simulink model "sm_potters_wheel"  (R2021b)
settings: Solver=ode15s  StartTime=0.0  StopTime=20  MaxStep=0.02  RelTol=1e-3  EnableMultiTasking=on
model workspace: external: MATLAB File sm_potters_wheel_params.m (data not in the file)
undefined symbols (not defined in the file or in its folder): actuation, clay, floor, leg, marker, shaft, sigbuilder_block, tabletop, wheel, X, Y, Z
libraries: sm_lib x48, nesl_utility x11
(part 1 of 2)
Description:
  | Sensing Composite Forces and Torques in Joints - Potter's Wheel
  | 
  | The example shows how you can sense forces and torques acting at joints. A
  | potter's wheel spins with a piecewise linear velocity profile while holding a piece
  | of clay off center. The clay creates a dynamic imbalance, generating periodic
  | constraint forces at the joints. Viscous damping accounts for energy dissipation
  | in the axle.
  | 
  | Scopes 1 and 2 show the composite forces and torques that you can sense at
  | the joints. These include the constraint forces and torques and also the total
  | forces and torques, which are the net sum of constraint, actuation and internal
  | components. The constraint components are zero in the direction of motion,
  | while the actuation and internal components are zero in the constrained directions.
  | 
  | If a multibody system is overconstrained, Simscape Multibody(TM) distributes the
  | constraint forces and torques over the joints enforcing the redundant constraints.
  | The vertical constraint forces acting at the leg weld joints are one example.
  | These forces, shown in Scope 3, add up to the total weight of the table. They
  | are nearly equal, with only slight discrepancies among them due to asymmetries
  | in the shape and position of the clay.
settings Model: Creator=The MathWorks, Inc.  LastModifiedBy=The MathWorks, Inc.
settings SolverCC: AlgebraicLoopSolver=TrustRegion
settings DataIOCC: LimitDataPoints=on  SaveFormat=Array  ReturnWorkspaceOutputs=off
settings OptimizationCC: LifeSpan=inf
settings DebuggingCC: SolverPrmCheckMsg=warning  SFUnexpectedBacktrackingDiag=warning  SFNoUnconditionalDefaultTransitionDiag=warning  SFExecutionAtInitializationDiag=none  SFMachineParentedDataDiag=warning  ArithmeticOperatorsInVariantConditions=warning
settings HardwareCC: ProdBitPerPointer=32  ProdBitPerSizeT=32  ProdBitPerPtrDiffT=32  ProdLargestAtomicFloat=None  ProdIntDivRoundTo=Undefined  ProdEndianess=Unspecified  ProdWordSize=32  ProdHWDeviceType=32-bit Generic
settings ModelReferenceCC: PropagateSignalLabelsOutOfModel=off
settings SFSimCC: SimUseLocalCustomCode=off  CustomCodeUndefinedFunction=UseInterfaceOnly
settings RTWCC: RTWUseLocalCustomCode=off
settings CodeAppCC: StateflowObjectComments=on
settings GRTTargetCC: TargetLangStandard=C89/C90 (ANSI)
settings ConfigComp: CovMetricSettings=dw  CovSaveCumulativeToWorkspaceVar=on  CovSaveSingleToWorkspaceVar=on  CovExternalEMLEnable=off  CovSFcnEnable=off
settings SimscapeCC: SimscapeNormalizeSystem=off
settings ConfigurationSet: Description=SimMechanics 2G
settings ExplorerConfigSet: InternalSimMechanicsExplorerSettings="<ExplorerConfiguration><canonicalview>default</canonicalview><AnimationSetting><BasePlaybackSpeed>1.0</BasePlaybackSpeed><PlaybackSpeedFactor>1.0</PlaybackSpeedFactor></AnimationSetting><TilePanel><TileInfo><Tiles Columns=\"1\" Count=\"1\" Rows=\"1\"><Column Left=\"2\" Weight=\"1\"/><Column Left=\"697\"/><Row Top=\"2\" Weight=\"1\"/><Row Top=\"673\"/><Tile Height=\"1\" Width=\"1\" X=\"0\" Y=\"0\"/></Tiles></TileInfo><SceneInfo><SceneViewer><BGColor><R>0.91372549533843994</R><G>0.92941176891326904</G><B>0.92941176891326904</B></BGColor><Camera><Position><X>1.1996229894546588</X><Y>-1.226238345212963</Y><Z>1.5340072938881431</Z></Position><Center><X>-0.0094998831543196653</X><Y>-0.017115472603984407</Y><Z>0.32488442127917233</Z></Center><Up><X>-0.40824829046386307</X><Y>0.40824829046386307</Y><Z>0.81649658092772615</Z></Up><Left>-0.60569783977149305</Left><Right>0.60569783977149305</Right><Bottom>-0.53853769779510163</Bottom><Top>0.53853769779510163</Top></Camera></SceneViewer></SceneInfo></TilePanel></ExplorerConfiguration>"

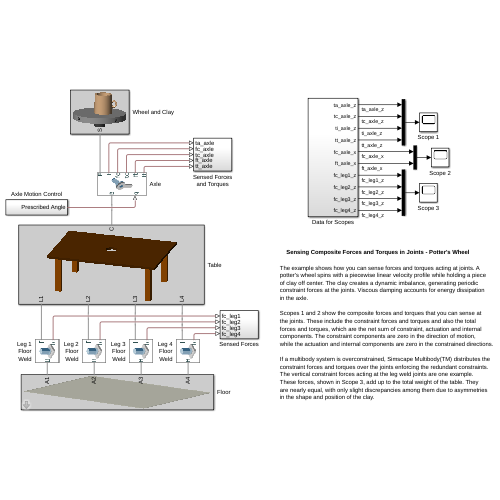
[thumbnail: Simulink's stored preview of the top-level diagram]
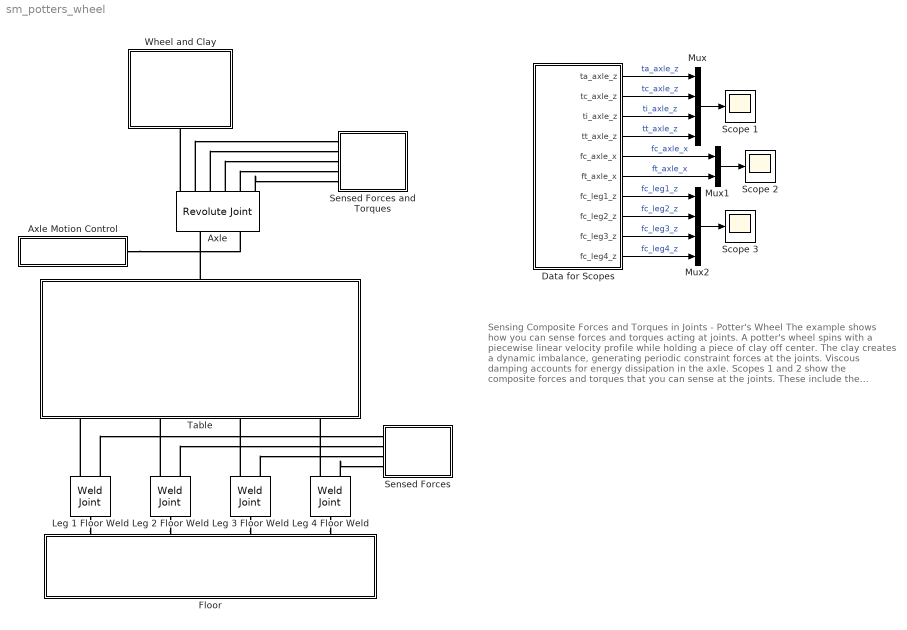
== system sm_potters_wheel ==
  note: Sensing Composite Forces and Torques in Joints - Potter's Wheel
      |
      | The example shows how you can sense forces and torques acting at joints. A
      | potter's wheel spins with a piecewise linear velocity profile while holding a piece
      | of clay off center. The clay creates a dynamic imbalance, generating periodic
      | constraint forces at the joints. Viscous damping accounts for energy dissipation
      | in the axle.
      |
      | Scopes 1 and 2 show the composite forces and torques that you can sense at
      | the joints. These include the constraint forces and torques and also the total
      | forces and torques, which are the net sum of constraint, actuation and internal
      | components. The constraint components are zero in the direction of motion,
      | while the actuation and internal components are zero in the constrained directions.
      |
      | If a multibody system is overconstrained, Simscape Multibody(TM) distributes the
      | constraint forces and torques over the joints enforcing the redundant constraints.
      | The vertical constraint forces acting at the leg weld joints are one example.
      | These forces, shown in Scope 3, add up to the total weight of the table. They
      | are nearly equal, with only slight discrepancies among them due to asymmetries
      | in the shape and position of the clay.
  Axle : sm_lib/Joints/Revolute Joint  JointMode=Normal  SenseConstraintForce=on  SenseConstraintForceX=off  SenseConstraintForceY=off  SenseConstraintForceZ=off  SenseConstraintTorque=on  SenseConstraintTorqueX=off  SenseConstraintTorqueY=off  SenseConstraintTorqueZ=off  SenseTotalForce=on  SenseTotalForceX=off  SenseTotalForceY=off  SenseTotalForceZ=off  SenseTotalTorque=on  SenseTotalTorqueX=off  SenseTotalTorqueY=off  SenseTotalTorqueZ=off  CompositeWrenchDir=BaseOnFollower  CompositeWrenchFrame=BaseFrame  EquilibriumPosition=0  EquilibriumPositionUnits=deg  SpringStiffness=0  SpringStiffnessUnits=N*m/deg  DampingCoefficient=axle.R.damping  DampingCoefficientUnits=N*m/(deg/s)  TorqueActuationMode=ComputedTorque  MotionActuationMode=InputMotion  SensePosition=off  SenseVelocity=off  SenseAcceleration=off  SenseTorqueForce=on  SenseLowerLimitTorqueForce=off  SenseUpperLimitTorqueForce=off  LowerLimitSpecify=off  LowerLimitBound=-90  LowerLimitBoundUnits=deg  LowerLimitStiffness=1e4  LowerLimitStiffnessUnits=N*m/deg  LowerLimitDamping=10  LowerLimitDampingUnits=N*m/(deg/s)  LowerLimitTransitionRegionWidth=0.1  LowerLimitTransitionRegionWidthUnits=deg  UpperLimitSpecify=off  UpperLimitBound=90  UpperLimitBoundUnits=deg  UpperLimitStiffness=1e4  UpperLimitStiffnessUnits=N*m/deg  UpperLimitDamping=10  UpperLimitDampingUnits=N*m/(deg/s)  UpperLimitTransitionRegionWidth=0.1  UpperLimitTransitionRegionWidthUnits=deg  PositionTargetSpecify=off  PositionTargetPriority=High  PositionTargetValue=0  PositionTargetValueUnits=deg  VelocityTargetSpecify=off  VelocityTargetPriority=High  VelocityTargetValue=0  VelocityTargetValueUnits=deg/s
  Axle Motion Control : Subsystem
  Data for Scopes : Subsystem
  Floor : Subsystem  mask(Floor){l=floor.length, w=floor.width, t=floor.thickness, la=tabletop.length - 2*tabletop.legoffset, wa=tabletop.width - 2*tabletop.legoffset, color=floor.color}
      mask prompts: l "Length (cm)"; w "Width (cm)"; t "Thickness (cm)"; la "Anchor Point Rectangle Length (cm)"; wa "Anchor Point Rectangle Width (cm)"; color "Color (RGB)"
      mask help:
      | This block models a floor for a table to stand on.
      |
      | Ports A1, A2, A3 and A4 correspond to four anchor frames on the upper plane of the floor. They lie at the corners of a rectangle aligned with the X and Y directions.
      mask init:
      | % Coordinates of anchor points
      | xa = la/2;
      | ya = wa/2;
      mask DialogControl Container4 Prompt: Dimensions
      mask DialogControl Container5 Prompt: Material Properties
      mask Display:
      | image(fullfile(matlabroot,'toolbox','physmod','sm','smdemos','potters_wheel','images','sm_pwheel_floor.png'));
      | port_label('RConn', 1, 'A1');
      | port_label('RConn', 2, 'A2');
      | port_label('RConn', 3, 'A3');
      | port_label('RConn', 4, 'A4');
  Leg 1 Floor Weld : sm_lib/Joints/Weld Joint  JointMode=Normal  SenseConstraintForce=on  SenseConstraintForceX=off  SenseConstraintForceY=off  SenseConstraintForceZ=off  SenseConstraintTorque=off  SenseConstraintTorqueX=off  SenseConstraintTorqueY=off  SenseConstraintTorqueZ=off  SenseTotalForce=off  SenseTotalForceX=off  SenseTotalForceY=off  SenseTotalForceZ=off  SenseTotalTorque=off  SenseTotalTorqueX=off  SenseTotalTorqueY=off  SenseTotalTorqueZ=off  CompositeWrenchDir=BaseOnFollower  CompositeWrenchFrame=BaseFrame
  Leg 2 Floor Weld : sm_lib/Joints/Weld Joint  JointMode=Normal  SenseConstraintForce=on  SenseConstraintForceX=off  SenseConstraintForceY=off  SenseConstraintForceZ=off  SenseConstraintTorque=off  SenseConstraintTorqueX=off  SenseConstraintTorqueY=off  SenseConstraintTorqueZ=off  SenseTotalForce=off  SenseTotalForceX=off  SenseTotalForceY=off  SenseTotalForceZ=off  SenseTotalTorque=off  SenseTotalTorqueX=off  SenseTotalTorqueY=off  SenseTotalTorqueZ=off  CompositeWrenchDir=BaseOnFollower  CompositeWrenchFrame=BaseFrame
  Leg 3 Floor Weld : sm_lib/Joints/Weld Joint  JointMode=Normal  SenseConstraintForce=on  SenseConstraintForceX=off  SenseConstraintForceY=off  SenseConstraintForceZ=off  SenseConstraintTorque=off  SenseConstraintTorqueX=off  SenseConstraintTorqueY=off  SenseConstraintTorqueZ=off  SenseTotalForce=off  SenseTotalForceX=off  SenseTotalForceY=off  SenseTotalForceZ=off  SenseTotalTorque=off  SenseTotalTorqueX=off  SenseTotalTorqueY=off  SenseTotalTorqueZ=off  CompositeWrenchDir=BaseOnFollower  CompositeWrenchFrame=BaseFrame
  Leg 4 Floor Weld : sm_lib/Joints/Weld Joint  JointMode=Normal  SenseConstraintForce=on  SenseConstraintForceX=off  SenseConstraintForceY=off  SenseConstraintForceZ=off  SenseConstraintTorque=off  SenseConstraintTorqueX=off  SenseConstraintTorqueY=off  SenseConstraintTorqueZ=off  SenseTotalForce=off  SenseTotalForceX=off  SenseTotalForceY=off  SenseTotalForceZ=off  SenseTotalTorque=off  SenseTotalTorqueX=off  SenseTotalTorqueY=off  SenseTotalTorqueZ=off  CompositeWrenchDir=BaseOnFollower  CompositeWrenchFrame=BaseFrame
  Mux : Mux
  Mux1 : Mux  Inputs=2
  Mux2 : Mux
  Scope 1 : Scope
  Scope 2 : Scope
  Scope 3 : Scope
  Sensed Forces : Subsystem
  Sensed Forces and Torques : Subsystem
  Table : Subsystem  mask(Table){}
      mask Display:
      | image(fullfile(matlabroot,'toolbox','physmod','sm','smdemos','potters_wheel','images','sm_pwheel_table.png'));
      | port_label('LConn', 1, 'L1')
      | port_label('LConn', 2, 'L2')
      | port_label('LConn', 3, 'L3')
      | port_label('LConn', 4, 'L4')
      | port_label('RConn', 1, 'C')
  Wheel and Clay : Subsystem  mask(Wheel and Clay){}
      mask Display:
      | image(fullfile(matlabroot,'toolbox','physmod','sm','smdemos','potters_wheel','images','sm_pwheel_wheelandclay.png'));
      | port_label('LConn', 1, 'S');
  wires:
  Mux/1 -> Scope 1/1
  Mux2/1 -> Scope 3/1
  Data for Scopes/1(ta_axle_z) -> Mux/1  "ta_axle_z"
  Data for Scopes/2(tc_axle_z) -> Mux/2  "tc_axle_z"
  Data for Scopes/3(ti_axle_z) -> Mux/3  "ti_axle_z"
  Data for Scopes/4(tt_axle_z) -> Mux/4  "tt_axle_z"
  Data for Scopes/5(fc_axle_x) -> Mux1/1  "fc_axle_x"
  Data for Scopes/6(ft_axle_x) -> Mux1/2  "ft_axle_x"
  Mux1/1 -> Scope 2/1
  Data for Scopes/8(fc_leg2_z) -> Mux2/2  "fc_leg2_z"
  Data for Scopes/9(fc_leg3_z) -> Mux2/3  "fc_leg3_z"
  Data for Scopes/10(fc_leg4_z) -> Mux2/4  "fc_leg4_z"
  Data for Scopes/7(fc_leg1_z) -> Mux2/1  "fc_leg1_z"
  connections:
  Axle/RConn1 -- Wheel and Clay/LConn1
  Table/RConn1 -- Axle/LConn1
  Axle Motion Control/RConn1 -- Axle/LConn2
  Axle/RConn6 -- Sensed Forces and Torques/LConn5
  Axle/RConn5 -- Sensed Forces and Torques/LConn4
  Axle/RConn4 -- Sensed Forces and Torques/LConn3
  Axle/RConn3 -- Sensed Forces and Torques/LConn2
  Axle/RConn2 -- Sensed Forces and Torques/LConn1
  Leg 1 Floor Weld/LConn1 -- Floor/RConn1
  Leg 1 Floor Weld/RConn1 -- Table/LConn1
  Leg 2 Floor Weld/LConn1 -- Floor/RConn2
  Leg 2 Floor Weld/RConn1 -- Table/LConn2
  Leg 3 Floor Weld/RConn1 -- Table/LConn3
  Leg 3 Floor Weld/LConn1 -- Floor/RConn3
  Leg 4 Floor Weld/RConn1 -- Table/LConn4
  Leg 4 Floor Weld/LConn1 -- Floor/RConn4
  Leg 4 Floor Weld/RConn2 -- Sensed Forces/LConn4
  Leg 3 Floor Weld/RConn2 -- Sensed Forces/LConn3
  Leg 2 Floor Weld/RConn2 -- Sensed Forces/LConn2
  Leg 1 Floor Weld/RConn2 -- Sensed Forces/LConn1

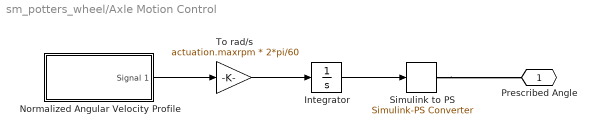
== system sm_potters_wheel/Axle Motion Control ==
  Integrator : Integrator
  Normalized Angular Velocity Profile : Subsystem  Tag=STV Subsys  LoadFcn=sigbuilder_block('load');  StartFcn=sigbuilder_block('start');  StopFcn=sigbuilder_block('stop');  ClipboardFcn=sigbuilder_block('clipboard');  mask(Sigbuilder block){tuvar=[0:10]}
      mask help: Simulink:masks:SigbuilderBlock_MD
      mask init:
      | if ~strcmp(get_param(bdroot(gcbh),'SimulationStatus'),'stopped') tuvar = sigbuilder_block('maskInit'); end
      settings: CopyFcn=sigbuilder_block('copy');  DeleteFcn=sigbuilder_block('delete');  ModelCloseFcn=sigbuilder_block('modelClose');  PreSaveFcn=sigbuilder_block('preSave');  PauseFcn=sigbuilder_block('pause');  ContinueFcn=sigbuilder_block('continue');  NameChangeFcn=sigbuilder_block('namechange');  OpenFcn=sigbuilder_block('open',[437.6 199.2 550.4 400 ]);  CloseFcn=sigbuilder_block('close');
      mask Display: plot(0, 0, 100, 100,[2, 2, 32, 32, 2], [68, 8, 8, 68, 68],[32, 2], [38, 38], [32, 19, 2],[53, 60, 44], [32, 17, 17, 2],[16, 16, 31, 31]);txt = getActiveGroup(gcbh);text(2, 100, txt,'verticalAlignment', 'top');
  Simulink to PS : nesl_utility/Simulink-PS Converter  PhysicalDomain=network_engine_domain  SubClassName=ps_input  LeftPortType=input  RightPortType=output  PseudoPeriodic=off  Frequencies=[]  NoiseDistribution=none  NoiseParameters=[]  Unit=rad  AffineConversion=off  FilteringAndDerivatives=filter  SimscapeFilterOrder=2  InputFilterTimeConstant=0.1  UdotUserProvided=1
      settings: SourceProductBaseCode=PW,SS
  To rad/s : Gain  Gain=actuation.maxrpm * 2*pi/60
  Prescribed Angle : PMIOPort  Side=Right
  wires:
  Normalized Angular Velocity Profile/1(Signal 1) -> To rad/s/1
  To rad/s/1 -> Integrator/1
  Integrator/1 -> Simulink to PS/1
  connections:
  Simulink to PS/RConn1 -- Prescribed Angle/RConn1

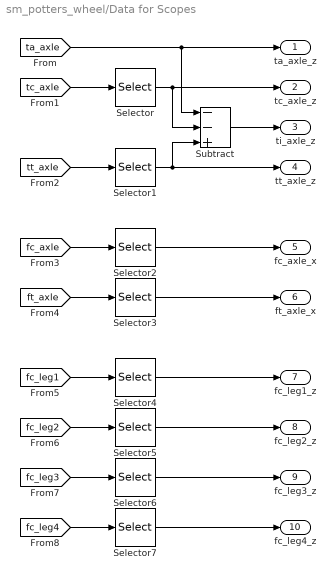
== system sm_potters_wheel/Data for Scopes ==
  Selector : Selector  InputPortWidth=3  IndexOptions=Index vector (dialog)  Indices=3  OutputSizes=1
  Selector1 : Selector  InputPortWidth=3  IndexOptions=Index vector (dialog)  Indices=3  OutputSizes=1
  Selector2 : Selector  InputPortWidth=3  IndexOptions=Index vector (dialog)  Indices=1  OutputSizes=1
  Selector3 : Selector  InputPortWidth=3  IndexOptions=Index vector (dialog)  Indices=1  OutputSizes=1
  Selector{4..7} (4 alike) : Selector  InputPortWidth=3  IndexOptions=Index vector (dialog)  Indices=3  OutputSizes=3
  Subtract : Sum  Inputs=--+
  ta_axle_z : Outport
  tc_axle_z : Outport  Port=2
  ti_axle_z : Outport  Port=3
  tt_axle_z : Outport  Port=4
  fc_axle_x : Outport  Port=5
  ft_axle_x : Outport  Port=6
  fc_leg1_z : Outport  Port=7
  fc_leg2_z : Outport  Port=8
  fc_leg3_z : Outport  Port=9
  fc_leg4_z : Outport  Port=10
  wires:
  [fc_leg1] -> Selector4/1
  [fc_axle] -> Selector2/1
  Selector/1 -> tc_axle_z/1, Subtract/2
  [tt_axle] -> Selector1/1
  [ft_axle] -> Selector3/1
  [tc_axle] -> Selector/1
  [ta_axle] -> ta_axle_z/1, Subtract/1
  Selector1/1 -> tt_axle_z/1, Subtract/3
  Subtract/1 -> ti_axle_z/1
  Selector4/1 -> fc_leg1_z/1
  Selector2/1 -> fc_axle_x/1
  Selector3/1 -> ft_axle_x/1
  [fc_leg2] -> Selector5/1
  Selector5/1 -> fc_leg2_z/1
  [fc_leg3] -> Selector6/1
  Selector6/1 -> fc_leg3_z/1
  [fc_leg4] -> Selector7/1
  Selector7/1 -> fc_leg4_z/1

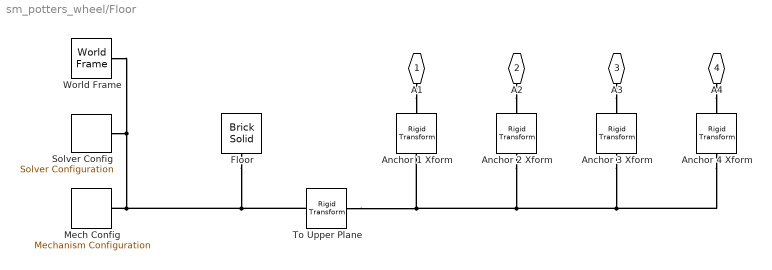
== system sm_potters_wheel/Floor ==
  Anchor 1 Xform : sm_lib/Frames and Transforms/Rigid Transform  TranslationMethod=Cartesian  TranslationStandardOffset=0  TranslationLengthUnit=cm  TranslationStandardAxis=+Z  TranslationCartesianOffset=[-xa ya 0]  TranslationROffset=0  TranslationROffsetUnits=m  TranslationZOffset=0  TranslationZOffsetUnits=m  TranslationThetaOffset=0  TranslationThetaOffsetUnits=deg  RotationMethod=None  RotationAngleUnits=deg  RotationStandardAxis=+Z  RotationAngle=0.0  RotationArbitraryAxis=[0 0 1]  FollAlignAxisA=+X  BaseAlignAxisA=+Y  FollAlignAxisB=+Y  BaseAlignAxisB=+Z  RotationSequenceAxes=FollowerAxes  RotationSequence=XYX  RotationSequenceAngles=[0 0 0]  RotationSequenceAnglesUnits=deg  RotationMatrix=[1 0 0; 0 1 0; 0 0 1]
  Anchor 2 Xform : sm_lib/Frames and Transforms/Rigid Transform  TranslationMethod=Cartesian  TranslationStandardOffset=0  TranslationLengthUnit=cm  TranslationStandardAxis=+Z  TranslationCartesianOffset=[-xa -ya 0]  TranslationROffset=0  TranslationROffsetUnits=m  TranslationZOffset=0  TranslationZOffsetUnits=m  TranslationThetaOffset=0  TranslationThetaOffsetUnits=deg  RotationMethod=None  RotationAngleUnits=deg  RotationStandardAxis=+Z  RotationAngle=0.0  RotationArbitraryAxis=[0 0 1]  FollAlignAxisA=+X  BaseAlignAxisA=+Y  FollAlignAxisB=+Y  BaseAlignAxisB=+Z  RotationSequenceAxes=FollowerAxes  RotationSequence=XYX  RotationSequenceAngles=[0 0 0]  RotationSequenceAnglesUnits=deg  RotationMatrix=[1 0 0; 0 1 0; 0 0 1]
  Anchor 3 Xform : sm_lib/Frames and Transforms/Rigid Transform  TranslationMethod=Cartesian  TranslationStandardOffset=0  TranslationLengthUnit=cm  TranslationStandardAxis=+Z  TranslationCartesianOffset=[xa -ya 0]  TranslationROffset=0  TranslationROffsetUnits=m  TranslationZOffset=0  TranslationZOffsetUnits=m  TranslationThetaOffset=0  TranslationThetaOffsetUnits=deg  RotationMethod=None  RotationAngleUnits=deg  RotationStandardAxis=+Z  RotationAngle=0.0  RotationArbitraryAxis=[0 0 1]  FollAlignAxisA=+X  BaseAlignAxisA=+Y  FollAlignAxisB=+Y  BaseAlignAxisB=+Z  RotationSequenceAxes=FollowerAxes  RotationSequence=XYX  RotationSequenceAngles=[0 0 0]  RotationSequenceAnglesUnits=deg  RotationMatrix=[1 0 0; 0 1 0; 0 0 1]
  Anchor 4 Xform : sm_lib/Frames and Transforms/Rigid Transform  TranslationMethod=Cartesian  TranslationStandardOffset=0  TranslationLengthUnit=cm  TranslationStandardAxis=+Z  TranslationCartesianOffset=[xa ya 0]  TranslationROffset=0  TranslationROffsetUnits=m  TranslationZOffset=0  TranslationZOffsetUnits=m  TranslationThetaOffset=0  TranslationThetaOffsetUnits=deg  RotationMethod=None  RotationAngleUnits=deg  RotationStandardAxis=+Z  RotationAngle=0.0  RotationArbitraryAxis=[0 0 1]  FollAlignAxisA=+X  BaseAlignAxisA=+Y  FollAlignAxisB=+Y  BaseAlignAxisB=+Z  RotationSequenceAxes=FollowerAxes  RotationSequence=XYX  RotationSequenceAngles=[0 0 0]  RotationSequenceAnglesUnits=deg  RotationMatrix=[1 0 0; 0 1 0; 0 0 1]
  Floor : sm_lib/Body Elements/Brick Solid  GraphicAmbientColor=[0.15 0.15 0.15 1.0]  BasedOnType=Density  BrickDimensions=[l w t]  BrickDimensionUnits=cm  CenterOfMass=[0 0 0]  CenterOfMassUnits=m  GraphicDiffuseColor=color  Density=1000  DensityUnits=kg/(m^3)  DoExposeReferenceFrame=on  GraphicEmissiveColor=[0.0 0.0 0.0 1.0]  ExportEntireGeometry=off  SerializedFrames=<Frames/>  MarkerShape=Sphere  MarkerSize=10  GraphicType=FromGeometry  InertiaType=PointMass  Mass=0  MassUnits=kg  MomentsOfInertia=[1 1 1]  MomentsOfInertiaUnits=kg*m^2  GraphicOpacity=0.5  ProductsOfInertia=[0 0 0]  ProductsOfInertiaUnits=kg*m^2  GraphicShininess=75  GraphicSpecularColor=[0.5 0.5 0.5 1.0]  GraphicVisPropType=SimpleVisualProperties
  Mech Config : sm_lib/Utilities/Mechanism Configuration  UniformGravity=Constant  GravityVector=[0 0 -9.80665]  GravityUnits=m/s^2  LinearizationDelta=0.001  JointModeTransitionNonlinearIterations=2
  Solver Config : nesl_utility/Solver Configuration  PhysicalDomain=network_engine_domain  SubClassName=solver  LeftPortType=input  RightPortType=generic  Tones=[]  Harmonics=[]  SimulateNoise=off  Profile=off  UseLocalSampling=off  EnableSwitchedLinearOptims=on  FrequencyDomain=off  UseCCode=off  RelTol=0.001  AbsTol=1e-06  MinStep=1e-09  ToWorkspace=off  RevertToSquareIcSolve=off  NumHomotopyIterations=100  PhasorMode=off  PhasorModeNumHarmonics=1  DoDC=off  ResidualTolerance=1e-09  UseLocalSolver=off  LocalSolverChoice=NE_BACKWARD_EULER_ADVANCER  LocalSolverSampleTime=0.001  DoFixedCost=off  MaxNonlinIter=3  MaxModeIter=2  ComputeImpulses=off  ImpulseIterations=2  LinearAlgebra=Sparse  EquationFormulation=NE_TIME_EF  DelaysMemoryBudget=1024  AutomaticFiltering=on  FilteringTimeConstant=0.001  PartitionStorageMethod=AS_NEEDED  PartitionMemoryBudget=1024  PartitionMethod=FAST
      settings: SourceProductBaseCode=PW,SS
  To Upper Plane : sm_lib/Frames and Transforms/Rigid Transform  TranslationMethod=Cartesian  TranslationStandardOffset=0  TranslationLengthUnit=cm  TranslationStandardAxis=+Z  TranslationCartesianOffset=[0 0 t/2]  TranslationROffset=0  TranslationROffsetUnits=m  TranslationZOffset=0  TranslationZOffsetUnits=m  TranslationThetaOffset=0  TranslationThetaOffsetUnits=deg  RotationMethod=None  RotationAngleUnits=deg  RotationStandardAxis=+Z  RotationAngle=0.0  RotationArbitraryAxis=[0 0 1]  FollAlignAxisA=+X  BaseAlignAxisA=+Y  FollAlignAxisB=+Y  BaseAlignAxisB=+Z  RotationSequenceAxes=FollowerAxes  RotationSequence=XYX  RotationSequenceAngles=[0 0 0]  RotationSequenceAnglesUnits=deg  RotationMatrix=[1 0 0; 0 1 0; 0 0 1]
  World Frame : sm_lib/Frames and Transforms/World Frame
  A1 : PMIOPort  Side=Right
  A2 : PMIOPort  Port=2  Side=Right
  A3 : PMIOPort  Port=3  Side=Right
  A4 : PMIOPort  Port=4  Side=Right
  connections:
  A2/RConn1 -- Anchor 2 Xform/RConn1
  A1/RConn1 -- Anchor 1 Xform/RConn1
  A3/RConn1 -- Anchor 3 Xform/RConn1
  A4/RConn1 -- Anchor 4 Xform/RConn1
  To Upper Plane/RConn1 -- Anchor 4 Xform/LConn1 -- Anchor 3 Xform/LConn1 -- Anchor 2 Xform/LConn1 -- Anchor 1 Xform/LConn1
  Solver Config/RConn1 -- Floor/RConn1 -- To Upper Plane/LConn1 -- Mech Config/RConn1 -- World Frame/RConn1

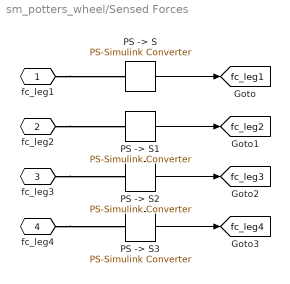
== system sm_potters_wheel/Sensed Forces ==
  PS -> S{,1..3} (4 alike) : nesl_utility/PS-Simulink Converter  PhysicalDomain=network_engine_domain  SubClassName=ps_output  LeftPortType=input  RightPortType=output  PseudoPeriodic=off  Frequencies=[]  Unit=N  AffineConversion=off
      settings: SourceProductBaseCode=PW,SS
  fc_leg1 : PMIOPort  Side=Left
  fc_leg2 : PMIOPort  Port=2  Side=Left
  fc_leg3 : PMIOPort  Port=3  Side=Left
  fc_leg4 : PMIOPort  Port=4  Side=Left
  tag scope: fc_leg1=global, fc_leg2=global, fc_leg3=global, fc_leg4=global
  wires:
  "PS -> S"/1 -> [fc_leg1]
  "PS -> S1"/1 -> [fc_leg2]
  "PS -> S2"/1 -> [fc_leg3]
  "PS -> S3"/1 -> [fc_leg4]
  connections:
  fc_leg1/RConn1 -- "PS -> S"/LConn1
  fc_leg2/RConn1 -- "PS -> S1"/LConn1
  fc_leg3/RConn1 -- "PS -> S2"/LConn1
  fc_leg4/RConn1 -- "PS -> S3"/LConn1

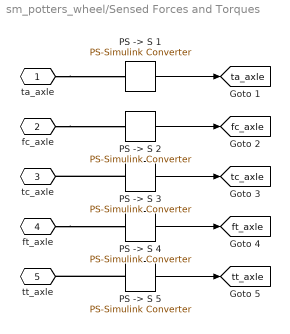
== system sm_potters_wheel/Sensed Forces and Torques ==
  "PS -> S 1" : nesl_utility/PS-Simulink Converter  PhysicalDomain=network_engine_domain  SubClassName=ps_output  LeftPortType=input  RightPortType=output  PseudoPeriodic=off  Frequencies=[]  Unit=N*m  AffineConversion=off
      settings: SourceProductBaseCode=PW,SS
  "PS -> S 2" : nesl_utility/PS-Simulink Converter  PhysicalDomain=network_engine_domain  SubClassName=ps_output  LeftPortType=input  RightPortType=output  PseudoPeriodic=off  Frequencies=[]  Unit=N  AffineConversion=off
      settings: SourceProductBaseCode=PW,SS
  "PS -> S 3" : nesl_utility/PS-Simulink Converter  PhysicalDomain=network_engine_domain  SubClassName=ps_output  LeftPortType=input  RightPortType=output  PseudoPeriodic=off  Frequencies=[]  Unit=N*m  AffineConversion=off
      settings: SourceProductBaseCode=PW,SS
  "PS -> S 4" : nesl_utility/PS-Simulink Converter  PhysicalDomain=network_engine_domain  SubClassName=ps_output  LeftPortType=input  RightPortType=output  PseudoPeriodic=off  Frequencies=[]  Unit=N  AffineConversion=off
      settings: SourceProductBaseCode=PW,SS
  "PS -> S 5" : nesl_utility/PS-Simulink Converter  PhysicalDomain=network_engine_domain  SubClassName=ps_output  LeftPortType=input  RightPortType=output  PseudoPeriodic=off  Frequencies=[]  Unit=N*m  AffineConversion=off
      settings: SourceProductBaseCode=PW,SS
  ta_axle : PMIOPort  Side=Left
  fc_axle : PMIOPort  Port=2  Side=Left
  tc_axle : PMIOPort  Port=3  Side=Left
  ft_axle : PMIOPort  Port=4  Side=Left
  tt_axle : PMIOPort  Port=5  Side=Left
  tag scope: fc_axle=global, ft_axle=global, ta_axle=global, tc_axle=global, tt_axle=global
  wires:
  "PS -> S 1"/1 -> [ta_axle]
  "PS -> S 3"/1 -> [tc_axle]
  "PS -> S 2"/1 -> [fc_axle]
  "PS -> S 5"/1 -> [tt_axle]
  "PS -> S 4"/1 -> [ft_axle]
  connections:
  "PS -> S 3"/LConn1 -- tc_axle/RConn1
  fc_axle/RConn1 -- "PS -> S 2"/LConn1
  ta_axle/RConn1 -- "PS -> S 1"/LConn1
  "PS -> S 5"/LConn1 -- tt_axle/RConn1
  ft_axle/RConn1 -- "PS -> S 4"/LConn1

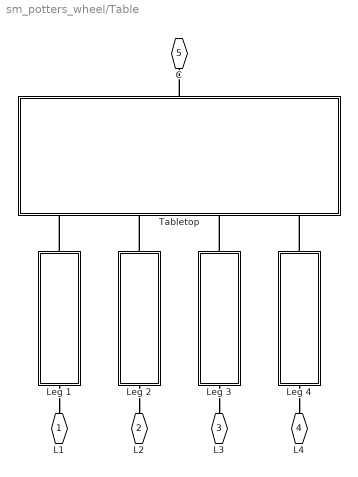
== system sm_potters_wheel/Table ==
  Leg 1 : Subsystem  mask(Table Leg){h=leg.height, w=leg.width, density=leg.density, color=leg.color}
      mask prompts: h "Leg Height (cm)"; w "Leg Width (cm)"; density "Density (kg/m^3)"; color "Color (RGB)"
      mask help:
      | This block models a straight table leg with square base.
      |
      | Port B corresponds to the frame at the base of the leg.
      |
      | Port T corresponds to the frame at the top of the leg.
      mask DialogControl Container4 Prompt: Dimensions
      mask DialogControl Container5 Prompt: Material Properties
      mask Display:
      | image(fullfile(matlabroot,'toolbox','physmod','sm','smdemos','potters_wheel','images','sm_pwheel_leg.png'));
      | port_label('LConn', 1, 'B');
      | port_label('RConn', 1, 'F');
  Leg 2 : Subsystem  mask(Table Leg){h=leg.height, w=leg.width, density=leg.density, color=leg.color}
      mask prompts: h "Leg Height (cm)"; w "Leg Width (cm)"; density "Density (kg/m^3)"; color "Color (RGB)"
      mask help:
      | This block models a straight table leg with square base.
      |
      | Port B corresponds to the frame at the base of the leg.
      |
      | Port T corresponds to the frame at the top of the leg.
      mask DialogControl Container4 Prompt: Dimensions
      mask DialogControl Container5 Prompt: Material Properties
      mask Display:
      | image(fullfile(matlabroot,'toolbox','physmod','sm','smdemos','potters_wheel','images','sm_pwheel_leg.png'));
      | port_label('LConn', 1, 'B');
      | port_label('RConn', 1, 'F');
  Leg 3 : Subsystem  mask(Table Leg){h=leg.height, w=leg.width, density=leg.density, color=leg.color}
      mask prompts: h "Leg Height (cm)"; w "Leg Width (cm)"; density "Density (kg/m^3)"; color "Color (RGB)"
      mask help:
      | This block models a straight table leg with square base.
      |
      | Port B corresponds to the frame at the base of the leg.
      |
      | Port T corresponds to the frame at the top of the leg.
      mask DialogControl Container4 Prompt: Dimensions
      mask DialogControl Container5 Prompt: Material Properties
      mask Display:
      | image(fullfile(matlabroot,'toolbox','physmod','sm','smdemos','potters_wheel','images','sm_pwheel_leg.png'));
      | port_label('LConn', 1, 'B');
      | port_label('RConn', 1, 'F');
  Leg 4 : Subsystem  mask(Table Leg){h=leg.height, w=leg.width, density=leg.density, color=leg.color}
      mask prompts: h "Leg Height (cm)"; w "Leg Width (cm)"; density "Density (kg/m^3)"; color "Color (RGB)"
      mask help:
      | This block models a straight table leg with square base.
      |
      | Port B corresponds to the frame at the base of the leg.
      |
      | Port T corresponds to the frame at the top of the leg.
      mask DialogControl Container4 Prompt: Dimensions
      mask DialogControl Container5 Prompt: Material Properties
      mask Display:
      | image(fullfile(matlabroot,'toolbox','physmod','sm','smdemos','potters_wheel','images','sm_pwheel_leg.png'));
      | port_label('LConn', 1, 'B');
      | port_label('RConn', 1, 'F');
  Tabletop : Subsystem  mask(Tabletop){a=tabletop.length, b=tabletop.width, r=tabletop.holeradius, t=tabletop.thickness, d=tabletop.legoffset, density=tabletop.density, color=tabletop.color}
      mask prompts: a "Length (cm)"; b "Width (cm)"; r "Center Hole Radius (cm)"; t "Thickness (cm)"; d "Leg Attachment Offset (cm)"; density "Density (kg/m^3)"; color "Color (RGB)"
      mask help:
      | This block models a flat rectangular tabletop, with a circular hole in the center to accommodate a cylindrical shaft.
      |
      | Ports L1, L2, L3 and L4 correspond to the frames at which the four legs are attached to the tabletop.
      |
      | Port C corresponds to the frame at the center of the tabletop.
      mask init:
      | %%%  Tabletop cross-section for extrusion
      | % Starting point
      | C0 = [  0   ,  b/2 ];
      | % Four corner points (in counter-clockwise order)
      | C1 = [ -a/2 ,  b/2 ];
      | C2 = [ -a/2 , -b/2 ];
      | C3 = [  a/2 , -b/2 ];
      | C4 = [  a/2 ,  b/2 ];
      | % Hole in the center (defined in the clockwise direction)
      | theta_cw = pi/180 * (450:-0.1:90)';
      | unit_circle_cw = [ cos(theta_cw) , sin(theta_cw) ];
      | H = r * unit_circle_cw;
      | % Build cross-section
      | section = [ C0 ; H ; C0 ; C1 ; C2 ; C3 ; C4 ];
      | 
      | %%%  Locations of leg attachment points (offset from corners)
      | L1 = C1 + [  d , -d ];
      | L2 = C2 + [  d ,  d ];
      | L3 = C3 + [ -d ,  d ];
      | L4 = C4 + [ -d , -d ];
      mask DialogControl Container4 Prompt: Dimensions
      mask DialogControl Container5 Prompt: Material Properties
      mask Display:
      | image(fullfile(matlabroot,'toolbox','physmod','sm','smdemos','potters_wheel','images','sm_pwheel_tabletop.png'));
      | port_label('LConn', 1, 'L1');
      | port_label('LConn', 2, 'L2');
      | port_label('LConn', 3, 'L3');
      | port_label('LConn', 4, 'L4');
      | port_label('RConn', 1, 'C');
  L1 : PMIOPort  Side=Left
  L2 : PMIOPort  Port=2  Side=Left
  L3 : PMIOPort  Port=3  Side=Left
  L4 : PMIOPort  Port=4  Side=Left
  C : PMIOPort  Port=5  Side=Right
  connections:
  Leg 1/LConn1 -- L1/RConn1
  Leg 2/LConn1 -- L2/RConn1
  Leg 3/LConn1 -- L3/RConn1
  Leg 4/LConn1 -- L4/RConn1
  Leg 3/RConn1 -- Tabletop/LConn3
  Leg 2/RConn1 -- Tabletop/LConn2
  Leg 1/RConn1 -- Tabletop/LConn1
  Leg 4/RConn1 -- Tabletop/LConn4
  Tabletop/RConn1 -- C/RConn1

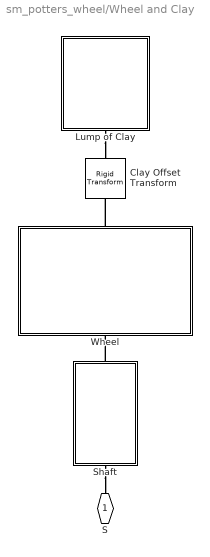
== system sm_potters_wheel/Wheel and Clay ==
  Clay Offset Transform : sm_lib/Frames and Transforms/Rigid Transform  TranslationMethod=StandardAxis  TranslationStandardOffset=clay.offset  TranslationLengthUnit=cm  TranslationStandardAxis=+X  TranslationCartesianOffset=[0 0 0]  TranslationROffset=0  TranslationROffsetUnits=m  TranslationZOffset=0  TranslationZOffsetUnits=m  TranslationThetaOffset=0  TranslationThetaOffsetUnits=deg  RotationMethod=None  RotationAngleUnits=deg  RotationStandardAxis=+Z  RotationAngle=0.0  RotationArbitraryAxis=[0 0 1]  FollAlignAxisA=+X  BaseAlignAxisA=+Y  FollAlignAxisB=+Y  BaseAlignAxisB=+Z  RotationSequenceAxes=FollowerAxes  RotationSequence=XYX  RotationSequenceAngles=[0 0 0]  RotationSequenceAnglesUnits=deg  RotationMatrix=[1 0 0; 0 1 0; 0 0 1]
  Lump of Clay : Subsystem  mask(Lump of Clay){h=clay.height, r=clay.radius, t=clay.thickness, rh=clay.handleradius, th=clay.handlethickness, density=clay.density, color=clay.color}
      mask prompts: h "Cup Height (cm)"; r "Cup Outer Radius (cm)"; t "Cup Thickness (cm)"; rh "Handle Radius (cm)"; th "Handle Thickness (cm)"; density "Density (kg/m^3)"; color "Color (RGB)"
      mask help:
      | This block models a lump of clay sitting on the potter's wheel. The clay has the form of a cup.
      |
      | Port C corresponds to the frame at the center of the bottom plane of the clay.
      mask init:
      | % L-shaped section for solid of revolution
      | % representing the clay cup
      | section_cup = [ ...
      |     r-t ,  h/2   ; ...
      |     r-t , -h/2+t ; ...
      |     0   , -h/2+t ; ...
      |     0   , -h/2   ; ...
      |     r   , -h/2   ; ...
      |     r   ,  h/2   ];
      | 
      | % Circular section for solid of revolution
      | % representing the cup's handle
      | theta = (0:1:360)'*pi/180;
      | section_handle = [ ...
      |     rh + th/2*cos(theta) , th/2*sin(theta) ];
      mask DialogControl Container4 Prompt: Dimensions
      mask DialogControl Container5 Prompt: Material Properties
      mask Display:
      | image(fullfile(matlabroot,'toolbox','physmod','sm','smdemos','potters_wheel','images','sm_pwheel_clay.png'));
      | port_label('LConn', 1, 'C');
  Shaft : Subsystem  mask(Shaft){h=shaft.length, r=shaft.radius, density=shaft.density, color=shaft.color}
      mask prompts: h "Length (cm)"; r "Radius (cm)"; density "Density (kg/m^3)"; color "Color (RGB)"
      mask help:
      | This block models a cylindrical shaft.
      |
      | Port S corresponds to the frame at the center of the shaft.
      |
      | Port T corresponds to the frame at the top of the shaft.
      mask DialogControl Container4 Prompt: Dimensions
      mask DialogControl Container5 Prompt: Material Properties
      mask Display:
      | image(fullfile(matlabroot,'toolbox','physmod','sm','smdemos','potters_wheel','images','sm_pwheel_shaft.png'));
      | port_label('LConn', 1, 'S');
      | port_label('RConn', 1, 'T');
  Wheel : Subsystem  mask(Wheel){h=wheel.thickness, r=wheel.radius, s=marker.size, density=wheel.density, color=wheel.color, c=marker.color}
      mask prompts: h "Thickness (cm)"; r "Radius (cm)"; s "Marker Size (cm)"; density "Density (kg/m^3)"; color "Color (RGB)"; c "Marker Color (RGB)"
      mask help:
      | This block models a circular wheel. Massless spherical markers on the perimeter help visualize the rotation of the wheel.
      |
      | Port B corresponds to the frame at the center of the bottom plane of the wheel.
      |
      | Port T corresponds to the frame at the center of the top plane of the wheel.
      mask DialogControl Container4 Prompt: Dimensions
      mask DialogControl Container5 Prompt: Material Properties
      mask Display:
      | image(fullfile(matlabroot,'toolbox','physmod','sm','smdemos','potters_wheel','images','sm_pwheel_wheel.png'));
      | port_label('LConn', 1, 'B');
      | port_label('RConn', 1, 'T');
  S : PMIOPort  Side=Left
  connections:
  Wheel/RConn1 -- Clay Offset Transform/LConn1
  Lump of Clay/LConn1 -- Clay Offset Transform/RConn1
  Shaft/RConn1 -- Wheel/LConn1
  Shaft/LConn1 -- S/RConn1

== system sm_potters_wheel/Axle Motion Control/Normalized Angular Velocity Profile ==
  Demux : Demux  Tag=STV Demux  Outputs=1
      settings: DisplayOption=none
  FromWs : FromWorkspace  Tag=STV FromWs  VariableName=tuvar
      SigBuilderData=|
      | common.afterFinalStr = 'Extrapolate'
      | common.sampleTime = 0
      | dataSet.timeRange = [0 20]
      | dataSet.name = 'Group 1'
      | sbobj.Groups.Name = 'Group 1'
      | sbobj.Groups.Signals.Name = 'Signal 1'
      | sbobj.Groups.Signals.XData = [0 1 1.2 6 10 15 20]
      | sbobj.Groups.Signals.YData = [0 0 0.2 0.2 1 1 0]
      | sbobj.Groups.TimeRange = [0 20]
  Signal 1 : Outport  Tag=STV Outport
  wires:
  Demux/1 -> Signal 1/1
  FromWs/1 -> Demux/1

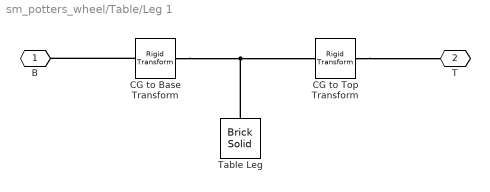
== system sm_potters_wheel/Table/Leg 1 ==
  CG to Base Transform : sm_lib/Frames and Transforms/Rigid Transform  TranslationMethod=StandardAxis  TranslationStandardOffset=h/2  TranslationLengthUnit=cm  TranslationStandardAxis=-Z  TranslationCartesianOffset=[0 0 0]  TranslationROffset=0  TranslationROffsetUnits=m  TranslationZOffset=0  TranslationZOffsetUnits=m  TranslationThetaOffset=0  TranslationThetaOffsetUnits=deg  RotationMethod=None  RotationAngleUnits=deg  RotationStandardAxis=+Z  RotationAngle=0.0  RotationArbitraryAxis=[0 0 1]  FollAlignAxisA=+X  BaseAlignAxisA=+Y  FollAlignAxisB=+Y  BaseAlignAxisB=+Z  RotationSequenceAxes=FollowerAxes  RotationSequence=XYX  RotationSequenceAngles=[0 0 0]  RotationSequenceAnglesUnits=deg  RotationMatrix=[1 0 0; 0 1 0; 0 0 1]
  CG to Top Transform : sm_lib/Frames and Transforms/Rigid Transform  TranslationMethod=StandardAxis  TranslationStandardOffset=h/2  TranslationLengthUnit=cm  TranslationStandardAxis=+Z  TranslationCartesianOffset=[0 0 0]  TranslationROffset=0  TranslationROffsetUnits=m  TranslationZOffset=0  TranslationZOffsetUnits=m  TranslationThetaOffset=0  TranslationThetaOffsetUnits=deg  RotationMethod=None  RotationAngleUnits=deg  RotationStandardAxis=+Z  RotationAngle=0.0  RotationArbitraryAxis=[0 0 1]  FollAlignAxisA=+X  BaseAlignAxisA=+Y  FollAlignAxisB=+Y  BaseAlignAxisB=+Z  RotationSequenceAxes=FollowerAxes  RotationSequence=XYX  RotationSequenceAngles=[0 0 0]  RotationSequenceAnglesUnits=deg  RotationMatrix=[1 0 0; 0 1 0; 0 0 1]
  Table Leg : sm_lib/Body Elements/Brick Solid  GraphicAmbientColor=[0.15 0.15 0.15 1.0]  BasedOnType=Density  BrickDimensions=[w w h]  BrickDimensionUnits=cm  CenterOfMass=[0 0 0]  CenterOfMassUnits=m  GraphicDiffuseColor=color  Density=density  DensityUnits=kg/(m^3)  DoExposeReferenceFrame=on  GraphicEmissiveColor=[0.0 0.0 0.0 1.0]  ExportEntireGeometry=off  SerializedFrames=<Frames/>  MarkerShape=Sphere  MarkerSize=10  GraphicType=FromGeometry  InertiaType=CalculateFromGeometry  Mass=1  MassUnits=kg  MomentsOfInertia=[1 1 1]  MomentsOfInertiaUnits=kg*m^2  GraphicOpacity=1.0  ProductsOfInertia=[0 0 0]  ProductsOfInertiaUnits=kg*m^2  GraphicShininess=75  GraphicSpecularColor=[0.5 0.5 0.5 1.0]  GraphicVisPropType=SimpleVisualProperties
  B : PMIOPort  Side=Left
  T : PMIOPort  Port=2  Side=Right
  connections:
  Table Leg/RConn1 -- CG to Base Transform/LConn1 -- CG to Top Transform/LConn1
  CG to Top Transform/RConn1 -- T/RConn1
  CG to Base Transform/RConn1 -- B/RConn1

== system sm_potters_wheel/Table/Leg 2 ==
  CG to Base Transform : sm_lib/Frames and Transforms/Rigid Transform  TranslationMethod=StandardAxis  TranslationStandardOffset=h/2  TranslationLengthUnit=cm  TranslationStandardAxis=-Z  TranslationCartesianOffset=[0 0 0]  TranslationROffset=0  TranslationROffsetUnits=m  TranslationZOffset=0  TranslationZOffsetUnits=m  TranslationThetaOffset=0  TranslationThetaOffsetUnits=deg  RotationMethod=None  RotationAngleUnits=deg  RotationStandardAxis=+Z  RotationAngle=0.0  RotationArbitraryAxis=[0 0 1]  FollAlignAxisA=+X  BaseAlignAxisA=+Y  FollAlignAxisB=+Y  BaseAlignAxisB=+Z  RotationSequenceAxes=FollowerAxes  RotationSequence=XYX  RotationSequenceAngles=[0 0 0]  RotationSequenceAnglesUnits=deg  RotationMatrix=[1 0 0; 0 1 0; 0 0 1]
  CG to Top Transform : sm_lib/Frames and Transforms/Rigid Transform  TranslationMethod=StandardAxis  TranslationStandardOffset=h/2  TranslationLengthUnit=cm  TranslationStandardAxis=+Z  TranslationCartesianOffset=[0 0 0]  TranslationROffset=0  TranslationROffsetUnits=m  TranslationZOffset=0  TranslationZOffsetUnits=m  TranslationThetaOffset=0  TranslationThetaOffsetUnits=deg  RotationMethod=None  RotationAngleUnits=deg  RotationStandardAxis=+Z  RotationAngle=0.0  RotationArbitraryAxis=[0 0 1]  FollAlignAxisA=+X  BaseAlignAxisA=+Y  FollAlignAxisB=+Y  BaseAlignAxisB=+Z  RotationSequenceAxes=FollowerAxes  RotationSequence=XYX  RotationSequenceAngles=[0 0 0]  RotationSequenceAnglesUnits=deg  RotationMatrix=[1 0 0; 0 1 0; 0 0 1]
  Table Leg : sm_lib/Body Elements/Brick Solid  GraphicAmbientColor=[0.15 0.15 0.15 1.0]  BasedOnType=Density  BrickDimensions=[w w h]  BrickDimensionUnits=cm  CenterOfMass=[0 0 0]  CenterOfMassUnits=m  GraphicDiffuseColor=color  Density=density  DensityUnits=kg/(m^3)  DoExposeReferenceFrame=on  GraphicEmissiveColor=[0.0 0.0 0.0 1.0]  ExportEntireGeometry=off  SerializedFrames=<Frames/>  MarkerShape=Sphere  MarkerSize=10  GraphicType=FromGeometry  InertiaType=CalculateFromGeometry  Mass=1  MassUnits=kg  MomentsOfInertia=[1 1 1]  MomentsOfInertiaUnits=kg*m^2  GraphicOpacity=1.0  ProductsOfInertia=[0 0 0]  ProductsOfInertiaUnits=kg*m^2  GraphicShininess=75  GraphicSpecularColor=[0.5 0.5 0.5 1.0]  GraphicVisPropType=SimpleVisualProperties
  B : PMIOPort  Side=Left
  T : PMIOPort  Port=2  Side=Right
  connections:
  CG to Base Transform/RConn1 -- B/RConn1
  CG to Top Transform/RConn1 -- T/RConn1
  CG to Top Transform/LConn1 -- CG to Base Transform/LConn1 -- Table Leg/RConn1

== system sm_potters_wheel/Table/Leg 3 ==
  CG to Base Transform : sm_lib/Frames and Transforms/Rigid Transform  TranslationMethod=StandardAxis  TranslationStandardOffset=h/2  TranslationLengthUnit=cm  TranslationStandardAxis=-Z  TranslationCartesianOffset=[0 0 0]  TranslationROffset=0  TranslationROffsetUnits=m  TranslationZOffset=0  TranslationZOffsetUnits=m  TranslationThetaOffset=0  TranslationThetaOffsetUnits=deg  RotationMethod=None  RotationAngleUnits=deg  RotationStandardAxis=+Z  RotationAngle=0.0  RotationArbitraryAxis=[0 0 1]  FollAlignAxisA=+X  BaseAlignAxisA=+Y  FollAlignAxisB=+Y  BaseAlignAxisB=+Z  RotationSequenceAxes=FollowerAxes  RotationSequence=XYX  RotationSequenceAngles=[0 0 0]  RotationSequenceAnglesUnits=deg  RotationMatrix=[1 0 0; 0 1 0; 0 0 1]
  CG to Top Transform : sm_lib/Frames and Transforms/Rigid Transform  TranslationMethod=StandardAxis  TranslationStandardOffset=h/2  TranslationLengthUnit=cm  TranslationStandardAxis=+Z  TranslationCartesianOffset=[0 0 0]  TranslationROffset=0  TranslationROffsetUnits=m  TranslationZOffset=0  TranslationZOffsetUnits=m  TranslationThetaOffset=0  TranslationThetaOffsetUnits=deg  RotationMethod=None  RotationAngleUnits=deg  RotationStandardAxis=+Z  RotationAngle=0.0  RotationArbitraryAxis=[0 0 1]  FollAlignAxisA=+X  BaseAlignAxisA=+Y  FollAlignAxisB=+Y  BaseAlignAxisB=+Z  RotationSequenceAxes=FollowerAxes  RotationSequence=XYX  RotationSequenceAngles=[0 0 0]  RotationSequenceAnglesUnits=deg  RotationMatrix=[1 0 0; 0 1 0; 0 0 1]
  Table Leg : sm_lib/Body Elements/Brick Solid  GraphicAmbientColor=[0.15 0.15 0.15 1.0]  BasedOnType=Density  BrickDimensions=[w w h]  BrickDimensionUnits=cm  CenterOfMass=[0 0 0]  CenterOfMassUnits=m  GraphicDiffuseColor=color  Density=density  DensityUnits=kg/(m^3)  DoExposeReferenceFrame=on  GraphicEmissiveColor=[0.0 0.0 0.0 1.0]  ExportEntireGeometry=off  SerializedFrames=<Frames/>  MarkerShape=Sphere  MarkerSize=10  GraphicType=FromGeometry  InertiaType=CalculateFromGeometry  Mass=1  MassUnits=kg  MomentsOfInertia=[1 1 1]  MomentsOfInertiaUnits=kg*m^2  GraphicOpacity=1.0  ProductsOfInertia=[0 0 0]  ProductsOfInertiaUnits=kg*m^2  GraphicShininess=75  GraphicSpecularColor=[0.5 0.5 0.5 1.0]  GraphicVisPropType=SimpleVisualProperties
  B : PMIOPort  Side=Left
  T : PMIOPort  Port=2  Side=Right
  connections:
  Table Leg/RConn1 -- CG to Base Transform/LConn1 -- CG to Top Transform/LConn1
  CG to Top Transform/RConn1 -- T/RConn1
  CG to Base Transform/RConn1 -- B/RConn1

== system sm_potters_wheel/Table/Leg 4 ==
  CG to Base Transform : sm_lib/Frames and Transforms/Rigid Transform  TranslationMethod=StandardAxis  TranslationStandardOffset=h/2  TranslationLengthUnit=cm  TranslationStandardAxis=-Z  TranslationCartesianOffset=[0 0 0]  TranslationROffset=0  TranslationROffsetUnits=m  TranslationZOffset=0  TranslationZOffsetUnits=m  TranslationThetaOffset=0  TranslationThetaOffsetUnits=deg  RotationMethod=None  RotationAngleUnits=deg  RotationStandardAxis=+Z  RotationAngle=0.0  RotationArbitraryAxis=[0 0 1]  FollAlignAxisA=+X  BaseAlignAxisA=+Y  FollAlignAxisB=+Y  BaseAlignAxisB=+Z  RotationSequenceAxes=FollowerAxes  RotationSequence=XYX  RotationSequenceAngles=[0 0 0]  RotationSequenceAnglesUnits=deg  RotationMatrix=[1 0 0; 0 1 0; 0 0 1]
  CG to Top Transform : sm_lib/Frames and Transforms/Rigid Transform  TranslationMethod=StandardAxis  TranslationStandardOffset=h/2  TranslationLengthUnit=cm  TranslationStandardAxis=+Z  TranslationCartesianOffset=[0 0 0]  TranslationROffset=0  TranslationROffsetUnits=m  TranslationZOffset=0  TranslationZOffsetUnits=m  TranslationThetaOffset=0  TranslationThetaOffsetUnits=deg  RotationMethod=None  RotationAngleUnits=deg  RotationStandardAxis=+Z  RotationAngle=0.0  RotationArbitraryAxis=[0 0 1]  FollAlignAxisA=+X  BaseAlignAxisA=+Y  FollAlignAxisB=+Y  BaseAlignAxisB=+Z  RotationSequenceAxes=FollowerAxes  RotationSequence=XYX  RotationSequenceAngles=[0 0 0]  RotationSequenceAnglesUnits=deg  RotationMatrix=[1 0 0; 0 1 0; 0 0 1]
  Table Leg : sm_lib/Body Elements/Brick Solid  GraphicAmbientColor=[0.15 0.15 0.15 1.0]  BasedOnType=Density  BrickDimensions=[w w h]  BrickDimensionUnits=cm  CenterOfMass=[0 0 0]  CenterOfMassUnits=m  GraphicDiffuseColor=color  Density=density  DensityUnits=kg/(m^3)  DoExposeReferenceFrame=on  GraphicEmissiveColor=[0.0 0.0 0.0 1.0]  ExportEntireGeometry=off  SerializedFrames=<Frames/>  MarkerShape=Sphere  MarkerSize=10  GraphicType=FromGeometry  InertiaType=CalculateFromGeometry  Mass=1  MassUnits=kg  MomentsOfInertia=[1 1 1]  MomentsOfInertiaUnits=kg*m^2  GraphicOpacity=1.0  ProductsOfInertia=[0 0 0]  ProductsOfInertiaUnits=kg*m^2  GraphicShininess=75  GraphicSpecularColor=[0.5 0.5 0.5 1.0]  GraphicVisPropType=SimpleVisualProperties
  B : PMIOPort  Side=Left
  T : PMIOPort  Port=2  Side=Right
  connections:
  CG to Base Transform/RConn1 -- B/RConn1
  CG to Top Transform/RConn1 -- T/RConn1
  CG to Top Transform/LConn1 -- CG to Base Transform/LConn1 -- Table Leg/RConn1

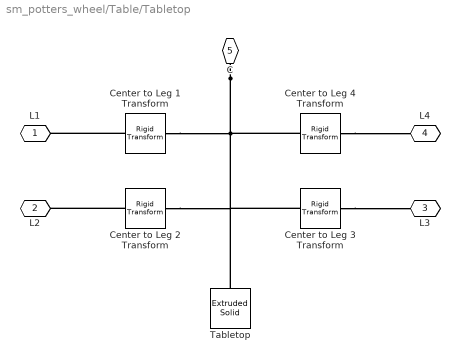
== system sm_potters_wheel/Table/Tabletop ==
  Center to Leg 1 Transform : sm_lib/Frames and Transforms/Rigid Transform  TranslationMethod=Cartesian  TranslationStandardOffset=0  TranslationLengthUnit=cm  TranslationStandardAxis=+Z  TranslationCartesianOffset=[L1 -t/2]  TranslationROffset=0  TranslationROffsetUnits=m  TranslationZOffset=0  TranslationZOffsetUnits=m  TranslationThetaOffset=0  TranslationThetaOffsetUnits=deg  RotationMethod=None  RotationAngleUnits=deg  RotationStandardAxis=+Z  RotationAngle=0.0  RotationArbitraryAxis=[0 0 1]  FollAlignAxisA=+X  BaseAlignAxisA=+Y  FollAlignAxisB=+Y  BaseAlignAxisB=+Z  RotationSequenceAxes=FollowerAxes  RotationSequence=XYX  RotationSequenceAngles=[0 0 0]  RotationSequenceAnglesUnits=deg  RotationMatrix=[1 0 0; 0 1 0; 0 0 1]
  Center to Leg 2 Transform : sm_lib/Frames and Transforms/Rigid Transform  TranslationMethod=Cartesian  TranslationStandardOffset=0  TranslationLengthUnit=cm  TranslationStandardAxis=+Z  TranslationCartesianOffset=[L2 -t/2]  TranslationROffset=0  TranslationROffsetUnits=m  TranslationZOffset=0  TranslationZOffsetUnits=m  TranslationThetaOffset=0  TranslationThetaOffsetUnits=deg  RotationMethod=None  RotationAngleUnits=deg  RotationStandardAxis=+Z  RotationAngle=0.0  RotationArbitraryAxis=[0 0 1]  FollAlignAxisA=+X  BaseAlignAxisA=+Y  FollAlignAxisB=+Y  BaseAlignAxisB=+Z  RotationSequenceAxes=FollowerAxes  RotationSequence=XYX  RotationSequenceAngles=[0 0 0]  RotationSequenceAnglesUnits=deg  RotationMatrix=[1 0 0; 0 1 0; 0 0 1]
  Center to Leg 3 Transform : sm_lib/Frames and Transforms/Rigid Transform  TranslationMethod=Cartesian  TranslationStandardOffset=0  TranslationLengthUnit=cm  TranslationStandardAxis=+Z  TranslationCartesianOffset=[L3 -t/2]  TranslationROffset=0  TranslationROffsetUnits=m  TranslationZOffset=0  TranslationZOffsetUnits=m  TranslationThetaOffset=0  TranslationThetaOffsetUnits=deg  RotationMethod=None  RotationAngleUnits=deg  RotationStandardAxis=+Z  RotationAngle=0.0  RotationArbitraryAxis=[0 0 1]  FollAlignAxisA=+X  BaseAlignAxisA=+Y  FollAlignAxisB=+Y  BaseAlignAxisB=+Z  RotationSequenceAxes=FollowerAxes  RotationSequence=XYX  RotationSequenceAngles=[0 0 0]  RotationSequenceAnglesUnits=deg  RotationMatrix=[1 0 0; 0 1 0; 0 0 1]
  Center to Leg 4 Transform : sm_lib/Frames and Transforms/Rigid Transform  TranslationMethod=Cartesian  TranslationStandardOffset=0  TranslationLengthUnit=cm  TranslationStandardAxis=+Z  TranslationCartesianOffset=[L4 -t/2]  TranslationROffset=0  TranslationROffsetUnits=m  TranslationZOffset=0  TranslationZOffsetUnits=m  TranslationThetaOffset=0  TranslationThetaOffsetUnits=deg  RotationMethod=None  RotationAngleUnits=deg  RotationStandardAxis=+Z  RotationAngle=0.0  RotationArbitraryAxis=[0 0 1]  FollAlignAxisA=+X  BaseAlignAxisA=+Y  FollAlignAxisB=+Y  BaseAlignAxisB=+Z  RotationSequenceAxes=FollowerAxes  RotationSequence=XYX  RotationSequenceAngles=[0 0 0]  RotationSequenceAnglesUnits=deg  RotationMatrix=[1 0 0; 0 1 0; 0 0 1]
  Tabletop : sm_lib/Body Elements/Extruded Solid  GraphicAmbientColor=[0.15 0.15 0.15 1.0]  BasedOnType=Density  CenterOfMass=[0 0 0]  CenterOfMassUnits=m  GraphicDiffuseColor=color  ExportConvexHullGeometry=off  ExtrusionCrossSection=section  ExtrusionCrossSectionUnits=cm  Density=density  DensityUnits=kg/(m^3)  DoExposeReferenceFrame=on  GraphicEmissiveColor=[0.0 0.0 0.0 1.0]  ExportEntireGeometry=off  ExtrusionLength=t  ExtrusionLengthUnits=cm  ExtrusionType=General  SerializedFrames=<Frames/>  MarkerShape=Sphere  MarkerSize=10  GraphicType=FromGeometry  InertiaType=CalculateFromGeometry  Mass=1  MassUnits=kg  MomentsOfInertia=[1 1 1]  MomentsOfInertiaUnits=kg*m^2  PolygonNumSides=3  GraphicOpacity=1.0  PolygonOuterRadius=1  PolygonOuterRadiusUnits=m  ProductsOfInertia=[0 0 0]  ProductsOfInertiaUnits=kg*m^2  GraphicShininess=75  GraphicSpecularColor=[0.5 0.5 0.5 1.0]  GraphicVisPropType=SimpleVisualProperties
  L1 : PMIOPort  Side=Left
  L2 : PMIOPort  Port=2  Side=Left
  L3 : PMIOPort  Port=3  Side=Left
  L4 : PMIOPort  Port=4  Side=Left
  C : PMIOPort  Port=5  Side=Right
  connections:
  C/RConn1 -- Tabletop/RConn1 -- Center to Leg 2 Transform/LConn1 -- Center to Leg 3 Transform/LConn1 -- Center to Leg 4 Transform/LConn1 -- Center to Leg 1 Transform/LConn1
  Center to Leg 4 Transform/RConn1 -- L4/RConn1
  Center to Leg 1 Transform/RConn1 -- L1/RConn1
  Center to Leg 3 Transform/RConn1 -- L3/RConn1
  Center to Leg 2 Transform/RConn1 -- L2/RConn1
